simulink model "distancesensor"  (R2019b)
settings: Solver=FixedStepAuto  StartTime=0.0  StopTime=999999  RelTol=1e-3  EnableMultiTasking=on
libraries: embdlinuxlib x6
settings Model: Creator=Vlad  LastModifiedBy=Vlad
settings SolverCC: PositivePriorityOrder=on
settings OptimizationCC: EnhancedBackFolding=on  PassReuseOutputArgsAs=Individual arguments  ZeroExternalMemoryAtStartup=off  ZeroInternalMemoryAtStartup=off  MaxStackSize=64  OptimizeBlockOrder=speed  DifferentSizesBufferReuse=on  OptimizationCustomize=off  EfficientTunableParamExpr=on
settings DebuggingCC: ParameterTunabilityLossMsg=error
settings HardwareCC: ProdBitPerPointer=32  ProdBitPerSizeT=32  ProdBitPerPtrDiffT=32  ProdLargestAtomicInteger=Long  ProdLargestAtomicFloat=Double  ProdWordSize=32  ProdLongLongMode=on  ProdHWDeviceType=ARM Compatible->ARM Cortex  UseEmbeddedCoderFeatures=off
settings RTWCC: SystemTargetFile=ert.tlc  HardwareBoard=Raspberry Pi  TLCOptions="-aInlineSetEventsForThisBaseRateFcn=TLC_FALSE -aSuppressMultiTaskScheduler=TLC_FALSE  -aRateBasedStepFcn=0"  TemplateMakefile=ert_default_tmf  GenerateReport=on  Toolchain=GNU GCC Raspberry Pi  BuildConfiguration=Faster Runs  IncludeHyperlinkInReport=on  LaunchReport=on  GenerateTraceInfo=on  GenerateTraceReport=on  GenerateTraceReportSl=on  GenerateTraceReportSf=on  GenerateTraceReportEml=on
settings CodeAppCC: ForceParamTrailComments=on  IgnoreCustomStorageClasses=off  OperatorAnnotations=on  SimulinkDataObjDesc=on  SFDataObjDesc=on  InsertBlockDesc=on
settings ERTTargetCC: SupportNonInlinedSFcns=on  SupportVariableSizeSignals=on

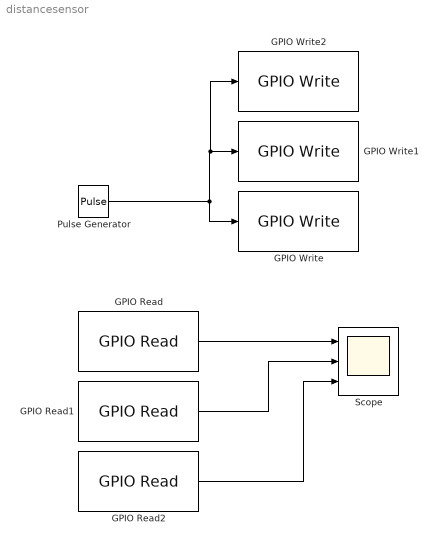
== system distancesensor ==
  GPIO Read : embdlinuxlib/GPIO Read  board=Pi Zero W  gpio=16  internalResistor=Off  sampleTime=0.0001  direction=Input  blockPlatform=Raspberry Pi
      settings: SourceProductName=Simulink Support Package for Raspberry Pi Hardware  SourceProductBaseCode=RASPPI
  GPIO Read1 : embdlinuxlib/GPIO Read  board=Pi Zero W  gpio=18  internalResistor=Off  sampleTime=0.0001  direction=Input  blockPlatform=Raspberry Pi
      settings: SourceProductName=Simulink Support Package for Raspberry Pi Hardware  SourceProductBaseCode=RASPPI
  GPIO Read2 : embdlinuxlib/GPIO Read  board=Pi Zero W  gpio=20  internalResistor=Off  sampleTime=0.0001  direction=Input  blockPlatform=Raspberry Pi
      settings: SourceProductName=Simulink Support Package for Raspberry Pi Hardware  SourceProductBaseCode=RASPPI
  GPIO Write : embdlinuxlib/GPIO Write  board=Pi Zero W  gpio=26  direction=Output  blockPlatform=Raspberry Pi
      settings: SourceProductName=Simulink Support Package for Raspberry Pi Hardware  SourceProductBaseCode=RASPPI
  GPIO Write1 : embdlinuxlib/GPIO Write  board=Pi Zero W  gpio=19  direction=Output  blockPlatform=Raspberry Pi
      settings: SourceProductName=Simulink Support Package for Raspberry Pi Hardware  SourceProductBaseCode=RASPPI
  GPIO Write2 : embdlinuxlib/GPIO Write  board=Pi Zero W  gpio=13  direction=Output  blockPlatform=Raspberry Pi
      settings: SourceProductName=Simulink Support Package for Raspberry Pi Hardware  SourceProductBaseCode=RASPPI
  Pulse Generator : DiscretePulseGenerator  PulseType=Time based  Period=1  PulseWidth=0.01
  Scope : Scope  NumInputPorts=3
  wires:
  Pulse Generator/1 -> GPIO Write/1, GPIO Write2/1, GPIO Write1/1
  GPIO Read/1 -> Scope/1
  GPIO Read1/1 -> Scope/2
  GPIO Read2/1 -> Scope/3
